simulink model "decimation"  (R2013b)
settings: Solver=ode45  StartTime=0.0  StopTime=10.0  RelTol=1e-3
undefined symbols (not defined in the file): xlfda_numerator
libraries: xbsIndex_r4 x1962, xps_library x2, casper_library_misc x1
(part 6 of 19)

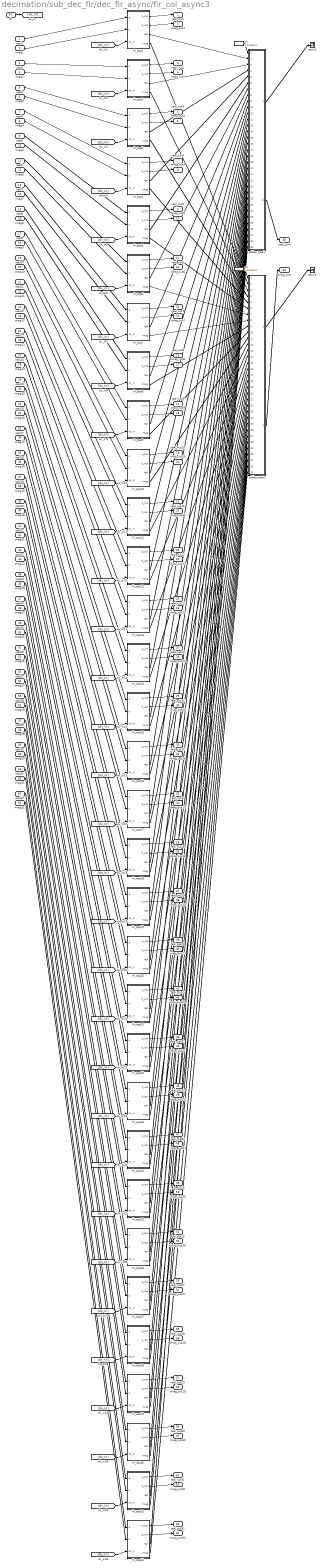
== system decimation/sub_dec_fir/dec_fir_async/fir_col_async3 ==
  real1 : Inport
  imag1 : Inport  Port=2
  real2 : Inport  Port=3
  imag2 : Inport  Port=4
  real3 : Inport  Port=5
  imag3 : Inport  Port=6
  real4 : Inport  Port=7
  imag4 : Inport  Port=8
  real5 : Inport  Port=9
  imag5 : Inport  Port=10
  real6 : Inport  Port=11
  imag6 : Inport  Port=12
  real7 : Inport  Port=13
  imag7 : Inport  Port=14
  real8 : Inport  Port=15
  imag8 : Inport  Port=16
  real9 : Inport  Port=17
  imag9 : Inport  Port=18
  real10 : Inport  Port=19
  imag10 : Inport  Port=20
  real11 : Inport  Port=21
  imag11 : Inport  Port=22
  real12 : Inport  Port=23
  imag12 : Inport  Port=24
  real13 : Inport  Port=25
  imag13 : Inport  Port=26
  real14 : Inport  Port=27
  imag14 : Inport  Port=28
  real15 : Inport  Port=29
  imag15 : Inport  Port=30
  real16 : Inport  Port=31
  imag16 : Inport  Port=32
  real17 : Inport  Port=33
  imag17 : Inport  Port=34
  real18 : Inport  Port=35
  imag18 : Inport  Port=36
  real19 : Inport  Port=37
  imag19 : Inport  Port=38
  real20 : Inport  Port=39
  imag20 : Inport  Port=40
  real21 : Inport  Port=41
  imag21 : Inport  Port=42
  real22 : Inport  Port=43
  imag22 : Inport  Port=44
  real23 : Inport  Port=45
  imag23 : Inport  Port=46
  real24 : Inport  Port=47
  imag24 : Inport  Port=48
  real25 : Inport  Port=49
  imag25 : Inport  Port=50
  real26 : Inport  Port=51
  imag26 : Inport  Port=52
  real27 : Inport  Port=53
  imag27 : Inport  Port=54
  real28 : Inport  Port=55
  imag28 : Inport  Port=56
  real29 : Inport  Port=57
  imag29 : Inport  Port=58
  real30 : Inport  Port=59
  imag30 : Inport  Port=60
  real31 : Inport  Port=61
  imag31 : Inport  Port=62
  real32 : Inport  Port=63
  imag32 : Inport  Port=64
  dv : Inport  Port=65
  adder_tree1 : Subsystem  AncestorBlock=casper_library_misc/adder_tree  mask(adder_tree){n_inputs=32, latency=1, adder_imp=DSP48, first_stage_hdl=on}
      mask prompts: n_inputs "Number of Inputs"; latency "Add Latency"; adder_imp "Adder implementation"; first_stage_hdl "Use behavioural HDL for first stage of adders"
      mask help:
      | Sums all inputs using a tree of adds and delays.
      |
      | Number of inputs: The number of inputs to the block to be summed
      | Add latency: The number of clock cycles to perform one addition (affects timing)..
      | Adder implementation: choice of fabric or DSP48E core, or behavioral HDL
      | Use behavioural HDL for first stage of adders: Causes the first stage of adders to be absorbed into DSP blocks if multipliers precede them (Virtex 5). Overrides Adder implementation
      mask init:
      | adder_tree_init(gcb, ...
      |     'n_inputs', n_inputs, ...
      |     'latency', latency, ...
      |     'adder_imp', adder_imp, ...
      |     'first_stage_hdl', first_stage_hdl);
      settings: AttributesFormatString=latency 5
      mask Help: eval('xlWeb(''http://casper.berkeley.edu/wiki/Adder_tree'')')
      mask TypeOptions adder_imp: Behavioral | Fabric | DSP48
  adder_tree2 : Subsystem  AncestorBlock=casper_library_misc/adder_tree  mask(adder_tree){n_inputs=32, latency=1, adder_imp=DSP48, first_stage_hdl=on}
      mask prompts: n_inputs "Number of Inputs"; latency "Add Latency"; adder_imp "Adder implementation"; first_stage_hdl "Use behavioural HDL for first stage of adders"
      mask help:
      | Sums all inputs using a tree of adds and delays.
      |
      | Number of inputs: The number of inputs to the block to be summed
      | Add latency: The number of clock cycles to perform one addition (affects timing)..
      | Adder implementation: choice of fabric or DSP48E core, or behavioral HDL
      | Use behavioural HDL for first stage of adders: Causes the first stage of adders to be absorbed into DSP blocks if multipliers precede them (Virtex 5). Overrides Adder implementation
      mask init:
      | adder_tree_init(gcb, ...
      |     'n_inputs', n_inputs, ...
      |     'latency', latency, ...
      |     'adder_imp', adder_imp, ...
      |     'first_stage_hdl', first_stage_hdl);
      settings: AttributesFormatString=latency 5
      mask Help: eval('xlWeb(''http://casper.berkeley.edu/wiki/Adder_tree'')')
      mask TypeOptions adder_imp: Behavioral | Fabric | DSP48
  c1 : xbsIndex_r4/Constant  const=1  gui_display_data_type=Fixed-point  arith_type=Signed (2's comp)  n_bits=16  bin_pt=14  preci_type=Single  exp_width=8  frac_width=24  explicit_period=on  period=1  equ=P=C  opselect=C  inp2=PCIN>>17  opr=+  inp1=P  carry=CIN  dbl_ovrd=off  block_type=constant
  c2 : xbsIndex_r4/Constant  const=1  gui_display_data_type=Fixed-point  arith_type=Signed (2's comp)  n_bits=16  bin_pt=14  preci_type=Single  exp_width=8  frac_width=24  explicit_period=on  period=1  equ=P=C  opselect=C  inp2=PCIN>>17  opr=+  inp1=P  carry=CIN  dbl_ovrd=off  block_type=constant
  fir_tap1 : Subsystem  AncestorBlock=casper_library_downconverter/fir_tap_async  mask(fir_tap_async){factor=-0.015819, add_latency=1, mult_latency=2, coeff_bit_width=25, coeff_bin_pt=24, async=on, dbl=off}
      mask prompts: add_latency "Add latency"; mult_latency "Mult latency"; coeff_bit_width "Coefficient bit width"; coeff_bin_pt "Coefficient binary point"; async "Asynchronous ops"; dbl "Double tap"
      mask help: Multiplies input data with factor specified.
      mask init:
      | fir_tap_async_init(gcb);
      mask Help: eval('xlWeb(''http://casper.berkeley.edu/wiki/Fir_tap'')')
  fir_tap10 : Subsystem  AncestorBlock=casper_library_downconverter/fir_tap_async  mask(fir_tap_async){factor=-0.0079781, add_latency=1, mult_latency=2, coeff_bit_width=25, coeff_bin_pt=24, async=on, dbl=off}
      mask prompts: add_latency "Add latency"; mult_latency "Mult latency"; coeff_bit_width "Coefficient bit width"; coeff_bin_pt "Coefficient binary point"; async "Asynchronous ops"; dbl "Double tap"
      mask help: Multiplies input data with factor specified.
      mask init:
      | fir_tap_async_init(gcb);
      mask Help: eval('xlWeb(''http://casper.berkeley.edu/wiki/Fir_tap'')')
  fir_tap11 : Subsystem  AncestorBlock=casper_library_downconverter/fir_tap_async  mask(fir_tap_async){factor=-0.0008307, add_latency=1, mult_latency=2, coeff_bit_width=25, coeff_bin_pt=24, async=on, dbl=off}
      mask prompts: add_latency "Add latency"; mult_latency "Mult latency"; coeff_bit_width "Coefficient bit width"; coeff_bin_pt "Coefficient binary point"; async "Asynchronous ops"; dbl "Double tap"
      mask help: Multiplies input data with factor specified.
      mask init:
      | fir_tap_async_init(gcb);
      mask Help: eval('xlWeb(''http://casper.berkeley.edu/wiki/Fir_tap'')')
  fir_tap12 : Subsystem  AncestorBlock=casper_library_downconverter/fir_tap_async  mask(fir_tap_async){factor=0.0066367, add_latency=1, mult_latency=2, coeff_bit_width=25, coeff_bin_pt=24, async=on, dbl=off}
      mask prompts: add_latency "Add latency"; mult_latency "Mult latency"; coeff_bit_width "Coefficient bit width"; coeff_bin_pt "Coefficient binary point"; async "Asynchronous ops"; dbl "Double tap"
      mask help: Multiplies input data with factor specified.
      mask init:
      | fir_tap_async_init(gcb);
      mask Help: eval('xlWeb(''http://casper.berkeley.edu/wiki/Fir_tap'')')
  fir_tap13 : Subsystem  AncestorBlock=casper_library_downconverter/fir_tap_async  mask(fir_tap_async){factor=0.0025836, add_latency=1, mult_latency=2, coeff_bit_width=25, coeff_bin_pt=24, async=on, dbl=off}
      mask prompts: add_latency "Add latency"; mult_latency "Mult latency"; coeff_bit_width "Coefficient bit width"; coeff_bin_pt "Coefficient binary point"; async "Asynchronous ops"; dbl "Double tap"
      mask help: Multiplies input data with factor specified.
      mask init:
      | fir_tap_async_init(gcb);
      mask Help: eval('xlWeb(''http://casper.berkeley.edu/wiki/Fir_tap'')')
  fir_tap14 : Subsystem  AncestorBlock=casper_library_downconverter/fir_tap_async  mask(fir_tap_async){factor=-0.0049848, add_latency=1, mult_latency=2, coeff_bit_width=25, coeff_bin_pt=24, async=on, dbl=off}
      mask prompts: add_latency "Add latency"; mult_latency "Mult latency"; coeff_bit_width "Coefficient bit width"; coeff_bin_pt "Coefficient binary point"; async "Asynchronous ops"; dbl "Double tap"
      mask help: Multiplies input data with factor specified.
      mask init:
      | fir_tap_async_init(gcb);
      mask Help: eval('xlWeb(''http://casper.berkeley.edu/wiki/Fir_tap'')')
  fir_tap15 : Subsystem  AncestorBlock=casper_library_downconverter/fir_tap_async  mask(fir_tap_async){factor=-0.0036243, add_latency=1, mult_latency=2, coeff_bit_width=25, coeff_bin_pt=24, async=on, dbl=off}
      mask prompts: add_latency "Add latency"; mult_latency "Mult latency"; coeff_bit_width "Coefficient bit width"; coeff_bin_pt "Coefficient binary point"; async "Asynchronous ops"; dbl "Double tap"
      mask help: Multiplies input data with factor specified.
      mask init:
      | fir_tap_async_init(gcb);
      mask Help: eval('xlWeb(''http://casper.berkeley.edu/wiki/Fir_tap'')')
  fir_tap16 : Subsystem  AncestorBlock=casper_library_downconverter/fir_tap_async  mask(fir_tap_async){factor=0.0032652, add_latency=1, mult_latency=2, coeff_bit_width=25, coeff_bin_pt=24, async=on, dbl=off}
      mask prompts: add_latency "Add latency"; mult_latency "Mult latency"; coeff_bit_width "Coefficient bit width"; coeff_bin_pt "Coefficient binary point"; async "Asynchronous ops"; dbl "Double tap"
      mask help: Multiplies input data with factor specified.
      mask init:
      | fir_tap_async_init(gcb);
      mask Help: eval('xlWeb(''http://casper.berkeley.edu/wiki/Fir_tap'')')
  fir_tap17 : Subsystem  AncestorBlock=casper_library_downconverter/fir_tap_async  mask(fir_tap_async){factor=0.0040292, add_latency=1, mult_latency=2, coeff_bit_width=25, coeff_bin_pt=24, async=on, dbl=off}
      mask prompts: add_latency "Add latency"; mult_latency "Mult latency"; coeff_bit_width "Coefficient bit width"; coeff_bin_pt "Coefficient binary point"; async "Asynchronous ops"; dbl "Double tap"
      mask help: Multiplies input data with factor specified.
      mask init:
      | fir_tap_async_init(gcb);
      mask Help: eval('xlWeb(''http://casper.berkeley.edu/wiki/Fir_tap'')')
  fir_tap18 : Subsystem  AncestorBlock=casper_library_downconverter/fir_tap_async  mask(fir_tap_async){factor=-0.0016691, add_latency=1, mult_latency=2, coeff_bit_width=25, coeff_bin_pt=24, async=on, dbl=off}
      mask prompts: add_latency "Add latency"; mult_latency "Mult latency"; coeff_bit_width "Coefficient bit width"; coeff_bin_pt "Coefficient binary point"; async "Asynchronous ops"; dbl "Double tap"
      mask help: Multiplies input data with factor specified.
      mask init:
      | fir_tap_async_init(gcb);
      mask Help: eval('xlWeb(''http://casper.berkeley.edu/wiki/Fir_tap'')')
  fir_tap19 : Subsystem  AncestorBlock=casper_library_downconverter/fir_tap_async  mask(fir_tap_async){factor=-0.0039196, add_latency=1, mult_latency=2, coeff_bit_width=25, coeff_bin_pt=24, async=on, dbl=off}
      mask prompts: add_latency "Add latency"; mult_latency "Mult latency"; coeff_bit_width "Coefficient bit width"; coeff_bin_pt "Coefficient binary point"; async "Asynchronous ops"; dbl "Double tap"
      mask help: Multiplies input data with factor specified.
      mask init:
      | fir_tap_async_init(gcb);
      mask Help: eval('xlWeb(''http://casper.berkeley.edu/wiki/Fir_tap'')')
  fir_tap2 : Subsystem  AncestorBlock=casper_library_downconverter/fir_tap_async  mask(fir_tap_async){factor=-0.0045283, add_latency=1, mult_latency=2, coeff_bit_width=25, coeff_bin_pt=24, async=on, dbl=off}
      mask prompts: add_latency "Add latency"; mult_latency "Mult latency"; coeff_bit_width "Coefficient bit width"; coeff_bin_pt "Coefficient binary point"; async "Asynchronous ops"; dbl "Double tap"
      mask help: Multiplies input data with factor specified.
      mask init:
      | fir_tap_async_init(gcb);
      mask Help: eval('xlWeb(''http://casper.berkeley.edu/wiki/Fir_tap'')')
  fir_tap20 : Subsystem  AncestorBlock=casper_library_downconverter/fir_tap_async  mask(fir_tap_async){factor=0.00032909, add_latency=1, mult_latency=2, coeff_bit_width=25, coeff_bin_pt=24, async=on, dbl=off}
      mask prompts: add_latency "Add latency"; mult_latency "Mult latency"; coeff_bit_width "Coefficient bit width"; coeff_bin_pt "Coefficient binary point"; async "Asynchronous ops"; dbl "Double tap"
      mask help: Multiplies input data with factor specified.
      mask init:
      | fir_tap_async_init(gcb);
      mask Help: eval('xlWeb(''http://casper.berkeley.edu/wiki/Fir_tap'')')
  fir_tap21 : Subsystem  AncestorBlock=casper_library_downconverter/fir_tap_async  mask(fir_tap_async){factor=0.0034399, add_latency=1, mult_latency=2, coeff_bit_width=25, coeff_bin_pt=24, async=on, dbl=off}
      mask prompts: add_latency "Add latency"; mult_latency "Mult latency"; coeff_bit_width "Coefficient bit width"; coeff_bin_pt "Coefficient binary point"; async "Asynchronous ops"; dbl "Double tap"
      mask help: Multiplies input data with factor specified.
      mask init:
      | fir_tap_async_init(gcb);
      mask Help: eval('xlWeb(''http://casper.berkeley.edu/wiki/Fir_tap'')')
  fir_tap22 : Subsystem  AncestorBlock=casper_library_downconverter/fir_tap_async  mask(fir_tap_async){factor=0.00068177, add_latency=1, mult_latency=2, coeff_bit_width=25, coeff_bin_pt=24, async=on, dbl=off}
      mask prompts: add_latency "Add latency"; mult_latency "Mult latency"; coeff_bit_width "Coefficient bit width"; coeff_bin_pt "Coefficient binary point"; async "Asynchronous ops"; dbl "Double tap"
      mask help: Multiplies input data with factor specified.
      mask init:
      | fir_tap_async_init(gcb);
      mask Help: eval('xlWeb(''http://casper.berkeley.edu/wiki/Fir_tap'')')
  fir_tap23 : Subsystem  AncestorBlock=casper_library_downconverter/fir_tap_async  mask(fir_tap_async){factor=-0.0027376, add_latency=1, mult_latency=2, coeff_bit_width=25, coeff_bin_pt=24, async=on, dbl=off}
      mask prompts: add_latency "Add latency"; mult_latency "Mult latency"; coeff_bit_width "Coefficient bit width"; coeff_bin_pt "Coefficient binary point"; async "Asynchronous ops"; dbl "Double tap"
      mask help: Multiplies input data with factor specified.
      mask init:
      | fir_tap_async_init(gcb);
      mask Help: eval('xlWeb(''http://casper.berkeley.edu/wiki/Fir_tap'')')
  fir_tap24 : Subsystem  AncestorBlock=casper_library_downconverter/fir_tap_async  mask(fir_tap_async){factor=-0.0013435, add_latency=1, mult_latency=2, coeff_bit_width=25, coeff_bin_pt=24, async=on, dbl=off}
      mask prompts: add_latency "Add latency"; mult_latency "Mult latency"; coeff_bit_width "Coefficient bit width"; coeff_bin_pt "Coefficient binary point"; async "Asynchronous ops"; dbl "Double tap"
      mask help: Multiplies input data with factor specified.
      mask init:
      | fir_tap_async_init(gcb);
      mask Help: eval('xlWeb(''http://casper.berkeley.edu/wiki/Fir_tap'')')
  fir_tap25 : Subsystem  AncestorBlock=casper_library_downconverter/fir_tap_async  mask(fir_tap_async){factor=0.0019468, add_latency=1, mult_latency=2, coeff_bit_width=25, coeff_bin_pt=24, async=on, dbl=off}
      mask prompts: add_latency "Add latency"; mult_latency "Mult latency"; coeff_bit_width "Coefficient bit width"; coeff_bin_pt "Coefficient binary point"; async "Asynchronous ops"; dbl "Double tap"
      mask help: Multiplies input data with factor specified.
      mask init:
      | fir_tap_async_init(gcb);
      mask Help: eval('xlWeb(''http://casper.berkeley.edu/wiki/Fir_tap'')')
  fir_tap26 : Subsystem  AncestorBlock=casper_library_downconverter/fir_tap_async  mask(fir_tap_async){factor=0.0016792, add_latency=1, mult_latency=2, coeff_bit_width=25, coeff_bin_pt=24, async=on, dbl=off}
      mask prompts: add_latency "Add latency"; mult_latency "Mult latency"; coeff_bit_width "Coefficient bit width"; coeff_bin_pt "Coefficient binary point"; async "Asynchronous ops"; dbl "Double tap"
      mask help: Multiplies input data with factor specified.
      mask init:
      | fir_tap_async_init(gcb);
      mask Help: eval('xlWeb(''http://casper.berkeley.edu/wiki/Fir_tap'')')
  fir_tap27 : Subsystem  AncestorBlock=casper_library_downconverter/fir_tap_async  mask(fir_tap_async){factor=-0.0011769, add_latency=1, mult_latency=2, coeff_bit_width=25, coeff_bin_pt=24, async=on, dbl=off}
      mask prompts: add_latency "Add latency"; mult_latency "Mult latency"; coeff_bit_width "Coefficient bit width"; coeff_bin_pt "Coefficient binary point"; async "Asynchronous ops"; dbl "Double tap"
      mask help: Multiplies input data with factor specified.
      mask init:
      | fir_tap_async_init(gcb);
      mask Help: eval('xlWeb(''http://casper.berkeley.edu/wiki/Fir_tap'')')
  fir_tap28 : Subsystem  AncestorBlock=casper_library_downconverter/fir_tap_async  mask(fir_tap_async){factor=-0.0017418, add_latency=1, mult_latency=2, coeff_bit_width=25, coeff_bin_pt=24, async=on, dbl=off}
      mask prompts: add_latency "Add latency"; mult_latency "Mult latency"; coeff_bit_width "Coefficient bit width"; coeff_bin_pt "Coefficient binary point"; async "Asynchronous ops"; dbl "Double tap"
      mask help: Multiplies input data with factor specified.
      mask init:
      | fir_tap_async_init(gcb);
      mask Help: eval('xlWeb(''http://casper.berkeley.edu/wiki/Fir_tap'')')
  fir_tap29 : Subsystem  AncestorBlock=casper_library_downconverter/fir_tap_async  mask(fir_tap_async){factor=0.00050609, add_latency=1, mult_latency=2, coeff_bit_width=25, coeff_bin_pt=24, async=on, dbl=off}
      mask prompts: add_latency "Add latency"; mult_latency "Mult latency"; coeff_bit_width "Coefficient bit width"; coeff_bin_pt "Coefficient binary point"; async "Asynchronous ops"; dbl "Double tap"
      mask help: Multiplies input data with factor specified.
      mask init:
      | fir_tap_async_init(gcb);
      mask Help: eval('xlWeb(''http://casper.berkeley.edu/wiki/Fir_tap'')')
  fir_tap3 : Subsystem  AncestorBlock=casper_library_downconverter/fir_tap_async  mask(fir_tap_async){factor=0.012178, add_latency=1, mult_latency=2, coeff_bit_width=25, coeff_bin_pt=24, async=on, dbl=off}
      mask prompts: add_latency "Add latency"; mult_latency "Mult latency"; coeff_bit_width "Coefficient bit width"; coeff_bin_pt "Coefficient binary point"; async "Asynchronous ops"; dbl "Double tap"
      mask help: Multiplies input data with factor specified.
      mask init:
      | fir_tap_async_init(gcb);
      mask Help: eval('xlWeb(''http://casper.berkeley.edu/wiki/Fir_tap'')')
  fir_tap30 : Subsystem  AncestorBlock=casper_library_downconverter/fir_tap_async  mask(fir_tap_async){factor=0.0016008, add_latency=1, mult_latency=2, coeff_bit_width=25, coeff_bin_pt=24, async=on, dbl=off}
      mask prompts: add_latency "Add latency"; mult_latency "Mult latency"; coeff_bit_width "Coefficient bit width"; coeff_bin_pt "Coefficient binary point"; async "Asynchronous ops"; dbl "Double tap"
      mask help: Multiplies input data with factor specified.
      mask init:
      | fir_tap_async_init(gcb);
      mask Help: eval('xlWeb(''http://casper.berkeley.edu/wiki/Fir_tap'')')
  fir_tap31 : Subsystem  AncestorBlock=casper_library_downconverter/fir_tap_async  mask(fir_tap_async){factor=1.9493e-05, add_latency=1, mult_latency=2, coeff_bit_width=25, coeff_bin_pt=24, async=on, dbl=off}
      mask prompts: add_latency "Add latency"; mult_latency "Mult latency"; coeff_bit_width "Coefficient bit width"; coeff_bin_pt "Coefficient binary point"; async "Asynchronous ops"; dbl "Double tap"
      mask help: Multiplies input data with factor specified.
      mask init:
      | fir_tap_async_init(gcb);
      mask Help: eval('xlWeb(''http://casper.berkeley.edu/wiki/Fir_tap'')')
  fir_tap32 : Subsystem  AncestorBlock=casper_library_downconverter/fir_tap_async  mask(fir_tap_async){factor=-0.0013302, add_latency=1, mult_latency=2, coeff_bit_width=25, coeff_bin_pt=24, async=on, dbl=off}
      mask prompts: add_latency "Add latency"; mult_latency "Mult latency"; coeff_bit_width "Coefficient bit width"; coeff_bin_pt "Coefficient binary point"; async "Asynchronous ops"; dbl "Double tap"
      mask help: Multiplies input data with factor specified.
      mask init:
      | fir_tap_async_init(gcb);
      mask Help: eval('xlWeb(''http://casper.berkeley.edu/wiki/Fir_tap'')')
  fir_tap4 : Subsystem  AncestorBlock=casper_library_downconverter/fir_tap_async  mask(fir_tap_async){factor=0.0072795, add_latency=1, mult_latency=2, coeff_bit_width=25, coeff_bin_pt=24, async=on, dbl=off}
      mask prompts: add_latency "Add latency"; mult_latency "Mult latency"; coeff_bit_width "Coefficient bit width"; coeff_bin_pt "Coefficient binary point"; async "Asynchronous ops"; dbl "Double tap"
      mask help: Multiplies input data with factor specified.
      mask init:
      | fir_tap_async_init(gcb);
      mask Help: eval('xlWeb(''http://casper.berkeley.edu/wiki/Fir_tap'')')
  fir_tap5 : Subsystem  AncestorBlock=casper_library_downconverter/fir_tap_async  mask(fir_tap_async){factor=-0.0083697, add_latency=1, mult_latency=2, coeff_bit_width=25, coeff_bin_pt=24, async=on, dbl=off}
      mask prompts: add_latency "Add latency"; mult_latency "Mult latency"; coeff_bit_width "Coefficient bit width"; coeff_bin_pt "Coefficient binary point"; async "Asynchronous ops"; dbl "Double tap"
      mask help: Multiplies input data with factor specified.
      mask init:
      | fir_tap_async_init(gcb);
      mask Help: eval('xlWeb(''http://casper.berkeley.edu/wiki/Fir_tap'')')
  fir_tap6 : Subsystem  AncestorBlock=casper_library_downconverter/fir_tap_async  mask(fir_tap_async){factor=-0.0085928, add_latency=1, mult_latency=2, coeff_bit_width=25, coeff_bin_pt=24, async=on, dbl=off}
      mask prompts: add_latency "Add latency"; mult_latency "Mult latency"; coeff_bit_width "Coefficient bit width"; coeff_bin_pt "Coefficient binary point"; async "Asynchronous ops"; dbl "Double tap"
      mask help: Multiplies input data with factor specified.
      mask init:
      | fir_tap_async_init(gcb);
      mask Help: eval('xlWeb(''http://casper.berkeley.edu/wiki/Fir_tap'')')
  fir_tap7 : Subsystem  AncestorBlock=casper_library_downconverter/fir_tap_async  mask(fir_tap_async){factor=0.004768, add_latency=1, mult_latency=2, coeff_bit_width=25, coeff_bin_pt=24, async=on, dbl=off}
      mask prompts: add_latency "Add latency"; mult_latency "Mult latency"; coeff_bit_width "Coefficient bit width"; coeff_bin_pt "Coefficient binary point"; async "Asynchronous ops"; dbl "Double tap"
      mask help: Multiplies input data with factor specified.
      mask init:
      | fir_tap_async_init(gcb);
      mask Help: eval('xlWeb(''http://casper.berkeley.edu/wiki/Fir_tap'')')
  fir_tap8 : Subsystem  AncestorBlock=casper_library_downconverter/fir_tap_async  mask(fir_tap_async){factor=0.008729, add_latency=1, mult_latency=2, coeff_bit_width=25, coeff_bin_pt=24, async=on, dbl=off}
      mask prompts: add_latency "Add latency"; mult_latency "Mult latency"; coeff_bit_width "Coefficient bit width"; coeff_bin_pt "Coefficient binary point"; async "Asynchronous ops"; dbl "Double tap"
      mask help: Multiplies input data with factor specified.
      mask init:
      | fir_tap_async_init(gcb);
      mask Help: eval('xlWeb(''http://casper.berkeley.edu/wiki/Fir_tap'')')
  fir_tap9 : Subsystem  AncestorBlock=casper_library_downconverter/fir_tap_async  mask(fir_tap_async){factor=-0.0016445, add_latency=1, mult_latency=2, coeff_bit_width=25, coeff_bin_pt=24, async=on, dbl=off}
      mask prompts: add_latency "Add latency"; mult_latency "Mult latency"; coeff_bit_width "Coefficient bit width"; coeff_bin_pt "Coefficient binary point"; async "Asynchronous ops"; dbl "Double tap"
      mask help: Multiplies input data with factor specified.
      mask init:
      | fir_tap_async_init(gcb);
      mask Help: eval('xlWeb(''http://casper.berkeley.edu/wiki/Fir_tap'')')
  term1 : Terminator
  term2 : Terminator
  real_out1 : Outport
  imag_out1 : Outport  Port=2
  real_out2 : Outport  Port=3
  imag_out2 : Outport  Port=4
  real_out3 : Outport  Port=5
  imag_out3 : Outport  Port=6
  real_out4 : Outport  Port=7
  imag_out4 : Outport  Port=8
  real_out5 : Outport  Port=9
  imag_out5 : Outport  Port=10
  real_out6 : Outport  Port=11
  imag_out6 : Outport  Port=12
  real_out7 : Outport  Port=13
  imag_out7 : Outport  Port=14
  real_out8 : Outport  Port=15
  imag_out8 : Outport  Port=16
  real_out9 : Outport  Port=17
  imag_out9 : Outport  Port=18
  real_out10 : Outport  Port=19
  imag_out10 : Outport  Port=20
  real_out11 : Outport  Port=21
  imag_out11 : Outport  Port=22
  real_out12 : Outport  Port=23
  imag_out12 : Outport  Port=24
  real_out13 : Outport  Port=25
  imag_out13 : Outport  Port=26
  real_out14 : Outport  Port=27
  imag_out14 : Outport  Port=28
  real_out15 : Outport  Port=29
  imag_out15 : Outport  Port=30
  real_out16 : Outport  Port=31
  imag_out16 : Outport  Port=32
  real_out17 : Outport  Port=33
  imag_out17 : Outport  Port=34
  real_out18 : Outport  Port=35
  imag_out18 : Outport  Port=36
  real_out19 : Outport  Port=37
  imag_out19 : Outport  Port=38
  real_out20 : Outport  Port=39
  imag_out20 : Outport  Port=40
  real_out21 : Outport  Port=41
  imag_out21 : Outport  Port=42
  real_out22 : Outport  Port=43
  imag_out22 : Outport  Port=44
  real_out23 : Outport  Port=45
  imag_out23 : Outport  Port=46
  real_out24 : Outport  Port=47
  imag_out24 : Outport  Port=48
  real_out25 : Outport  Port=49
  imag_out25 : Outport  Port=50
  real_out26 : Outport  Port=51
  imag_out26 : Outport  Port=52
  real_out27 : Outport  Port=53
  imag_out27 : Outport  Port=54
  real_out28 : Outport  Port=55
  imag_out28 : Outport  Port=56
  real_out29 : Outport  Port=57
  imag_out29 : Outport  Port=58
  real_out30 : Outport  Port=59
  imag_out30 : Outport  Port=60
  real_out31 : Outport  Port=61
  imag_out31 : Outport  Port=62
  real_out32 : Outport  Port=63
  imag_out32 : Outport  Port=64
  real_sum : Outport  Port=65
  imag_sum : Outport  Port=66
  wires:
  dv/1 -> [dv_in]
  [dv_in] -> fir_tap1/3(dv_in)
  real1/1 -> fir_tap1/1(a)
  imag1/1 -> fir_tap1/2(b)
  [dv_in] -> fir_tap2/3(dv_in)
  real2/1 -> fir_tap2/1(a)
  imag2/1 -> fir_tap2/2(b)
  [dv_in] -> fir_tap3/3(dv_in)
  real3/1 -> fir_tap3/1(a)
  imag3/1 -> fir_tap3/2(b)
  [dv_in] -> fir_tap4/3(dv_in)
  real4/1 -> fir_tap4/1(a)
  imag4/1 -> fir_tap4/2(b)
  [dv_in] -> fir_tap5/3(dv_in)
  real5/1 -> fir_tap5/1(a)
  imag5/1 -> fir_tap5/2(b)
  [dv_in] -> fir_tap6/3(dv_in)
  real6/1 -> fir_tap6/1(a)
  imag6/1 -> fir_tap6/2(b)
  [dv_in] -> fir_tap7/3(dv_in)
  real7/1 -> fir_tap7/1(a)
  imag7/1 -> fir_tap7/2(b)
  [dv_in] -> fir_tap8/3(dv_in)
  real8/1 -> fir_tap8/1(a)
  imag8/1 -> fir_tap8/2(b)
  [dv_in] -> fir_tap9/3(dv_in)
  real9/1 -> fir_tap9/1(a)
  imag9/1 -> fir_tap9/2(b)
  [dv_in] -> fir_tap10/3(dv_in)
  real10/1 -> fir_tap10/1(a)
  imag10/1 -> fir_tap10/2(b)
  [dv_in] -> fir_tap11/3(dv_in)
  real11/1 -> fir_tap11/1(a)
  imag11/1 -> fir_tap11/2(b)
  [dv_in] -> fir_tap12/3(dv_in)
  real12/1 -> fir_tap12/1(a)
  imag12/1 -> fir_tap12/2(b)
  [dv_in] -> fir_tap13/3(dv_in)
  real13/1 -> fir_tap13/1(a)
  imag13/1 -> fir_tap13/2(b)
  [dv_in] -> fir_tap14/3(dv_in)
  real14/1 -> fir_tap14/1(a)
  imag14/1 -> fir_tap14/2(b)
  [dv_in] -> fir_tap15/3(dv_in)
  real15/1 -> fir_tap15/1(a)
  imag15/1 -> fir_tap15/2(b)
  [dv_in] -> fir_tap16/3(dv_in)
  real16/1 -> fir_tap16/1(a)
  imag16/1 -> fir_tap16/2(b)
  [dv_in] -> fir_tap17/3(dv_in)
  real17/1 -> fir_tap17/1(a)
  imag17/1 -> fir_tap17/2(b)
  [dv_in] -> fir_tap18/3(dv_in)
  real18/1 -> fir_tap18/1(a)
  imag18/1 -> fir_tap18/2(b)
  [dv_in] -> fir_tap19/3(dv_in)
  real19/1 -> fir_tap19/1(a)
  imag19/1 -> fir_tap19/2(b)
  [dv_in] -> fir_tap20/3(dv_in)
  real20/1 -> fir_tap20/1(a)
  imag20/1 -> fir_tap20/2(b)
  [dv_in] -> fir_tap21/3(dv_in)
  real21/1 -> fir_tap21/1(a)
  imag21/1 -> fir_tap21/2(b)
  [dv_in] -> fir_tap22/3(dv_in)
  real22/1 -> fir_tap22/1(a)
  imag22/1 -> fir_tap22/2(b)
  [dv_in] -> fir_tap23/3(dv_in)
  real23/1 -> fir_tap23/1(a)
  imag23/1 -> fir_tap23/2(b)
  [dv_in] -> fir_tap24/3(dv_in)
  real24/1 -> fir_tap24/1(a)
  imag24/1 -> fir_tap24/2(b)
  [dv_in] -> fir_tap25/3(dv_in)
  real25/1 -> fir_tap25/1(a)
  imag25/1 -> fir_tap25/2(b)
  [dv_in] -> fir_tap26/3(dv_in)
  real26/1 -> fir_tap26/1(a)
  imag26/1 -> fir_tap26/2(b)
  [dv_in] -> fir_tap27/3(dv_in)
  real27/1 -> fir_tap27/1(a)
  imag27/1 -> fir_tap27/2(b)
  [dv_in] -> fir_tap28/3(dv_in)
  real28/1 -> fir_tap28/1(a)
  imag28/1 -> fir_tap28/2(b)
  [dv_in] -> fir_tap29/3(dv_in)
  real29/1 -> fir_tap29/1(a)
  imag29/1 -> fir_tap29/2(b)
  [dv_in] -> fir_tap30/3(dv_in)
  real30/1 -> fir_tap30/1(a)
  imag30/1 -> fir_tap30/2(b)
  [dv_in] -> fir_tap31/3(dv_in)
  real31/1 -> fir_tap31/1(a)
  imag31/1 -> fir_tap31/2(b)
  [dv_in] -> fir_tap32/3(dv_in)
  real32/1 -> fir_tap32/1(a)
  imag32/1 -> fir_tap32/2(b)
  fir_tap1/1(a_out) -> real_out1/1
  fir_tap1/2(b_out) -> imag_out1/1
  fir_tap2/1(a_out) -> real_out2/1
  fir_tap2/2(b_out) -> imag_out2/1
  fir_tap3/1(a_out) -> real_out3/1
  fir_tap3/2(b_out) -> imag_out3/1
  fir_tap4/1(a_out) -> real_out4/1
  fir_tap4/2(b_out) -> imag_out4/1
  fir_tap5/1(a_out) -> real_out5/1
  fir_tap5/2(b_out) -> imag_out5/1
  fir_tap6/1(a_out) -> real_out6/1
  fir_tap6/2(b_out) -> imag_out6/1
  fir_tap7/1(a_out) -> real_out7/1
  fir_tap7/2(b_out) -> imag_out7/1
  fir_tap8/1(a_out) -> real_out8/1
  fir_tap8/2(b_out) -> imag_out8/1
  fir_tap9/1(a_out) -> real_out9/1
  fir_tap9/2(b_out) -> imag_out9/1
  fir_tap10/1(a_out) -> real_out10/1
  fir_tap10/2(b_out) -> imag_out10/1
  fir_tap11/1(a_out) -> real_out11/1
  fir_tap11/2(b_out) -> imag_out11/1
  fir_tap12/1(a_out) -> real_out12/1
  fir_tap12/2(b_out) -> imag_out12/1
  fir_tap13/1(a_out) -> real_out13/1
  fir_tap13/2(b_out) -> imag_out13/1
  fir_tap14/1(a_out) -> real_out14/1
  fir_tap14/2(b_out) -> imag_out14/1
  fir_tap15/1(a_out) -> real_out15/1
  fir_tap15/2(b_out) -> imag_out15/1
  fir_tap16/1(a_out) -> real_out16/1
  fir_tap16/2(b_out) -> imag_out16/1
  fir_tap17/1(a_out) -> real_out17/1
  fir_tap17/2(b_out) -> imag_out17/1
  fir_tap18/1(a_out) -> real_out18/1
  fir_tap18/2(b_out) -> imag_out18/1
  fir_tap19/1(a_out) -> real_out19/1
  fir_tap19/2(b_out) -> imag_out19/1
  fir_tap20/1(a_out) -> real_out20/1
  fir_tap20/2(b_out) -> imag_out20/1
  fir_tap21/1(a_out) -> real_out21/1
  fir_tap21/2(b_out) -> imag_out21/1
  fir_tap22/1(a_out) -> real_out22/1
  fir_tap22/2(b_out) -> imag_out22/1
  fir_tap23/1(a_out) -> real_out23/1
  fir_tap23/2(b_out) -> imag_out23/1
  fir_tap24/1(a_out) -> real_out24/1
  fir_tap24/2(b_out) -> imag_out24/1
  fir_tap25/1(a_out) -> real_out25/1
  fir_tap25/2(b_out) -> imag_out25/1
  fir_tap26/1(a_out) -> real_out26/1
  fir_tap26/2(b_out) -> imag_out26/1
  fir_tap27/1(a_out) -> real_out27/1
  fir_tap27/2(b_out) -> imag_out27/1
  fir_tap28/1(a_out) -> real_out28/1
  fir_tap28/2(b_out) -> imag_out28/1
  fir_tap29/1(a_out) -> real_out29/1
  fir_tap29/2(b_out) -> imag_out29/1
  fir_tap30/1(a_out) -> real_out30/1
  fir_tap30/2(b_out) -> imag_out30/1
  fir_tap31/1(a_out) -> real_out31/1
  fir_tap31/2(b_out) -> imag_out31/1
  fir_tap32/1(a_out) -> real_out32/1
  fir_tap32/2(b_out) -> imag_out32/1
  adder_tree1/1(sync_out) -> term1/1
  adder_tree2/1(sync_out) -> term2/1
  c1/1 -> adder_tree1/1(sync)
  c2/1 -> adder_tree2/1(sync)
  adder_tree1/2(dout) -> real_sum/1
  adder_tree2/2(dout) -> imag_sum/1
  fir_tap1/3(real) -> adder_tree1/2(din1)
  fir_tap1/4(imag) -> adder_tree2/2(din1)
  fir_tap2/3(real) -> adder_tree1/3(din2)
  fir_tap2/4(imag) -> adder_tree2/3(din2)
  fir_tap3/3(real) -> adder_tree1/4(din3)
  fir_tap3/4(imag) -> adder_tree2/4(din3)
  fir_tap4/3(real) -> adder_tree1/5(din4)
  fir_tap4/4(imag) -> adder_tree2/5(din4)
  fir_tap5/3(real) -> adder_tree1/6(din5)
  fir_tap5/4(imag) -> adder_tree2/6(din5)
  fir_tap6/3(real) -> adder_tree1/7(din6)
  fir_tap6/4(imag) -> adder_tree2/7(din6)
  fir_tap7/3(real) -> adder_tree1/8(din7)
  fir_tap7/4(imag) -> adder_tree2/8(din7)
  fir_tap8/3(real) -> adder_tree1/9(din8)
  fir_tap8/4(imag) -> adder_tree2/9(din8)
  fir_tap9/3(real) -> adder_tree1/10(din9)
  fir_tap9/4(imag) -> adder_tree2/10(din9)
  fir_tap10/3(real) -> adder_tree1/11(din10)
  fir_tap10/4(imag) -> adder_tree2/11(din10)
  fir_tap11/3(real) -> adder_tree1/12(din11)
  fir_tap11/4(imag) -> adder_tree2/12(din11)
  fir_tap12/3(real) -> adder_tree1/13(din12)
  fir_tap12/4(imag) -> adder_tree2/13(din12)
  fir_tap13/3(real) -> adder_tree1/14(din13)
  fir_tap13/4(imag) -> adder_tree2/14(din13)
  fir_tap14/3(real) -> adder_tree1/15(din14)
  fir_tap14/4(imag) -> adder_tree2/15(din14)
  fir_tap15/3(real) -> adder_tree1/16(din15)
  fir_tap15/4(imag) -> adder_tree2/16(din15)
  fir_tap16/3(real) -> adder_tree1/17(din16)
  fir_tap16/4(imag) -> adder_tree2/17(din16)
  fir_tap17/3(real) -> adder_tree1/18(din17)
  fir_tap17/4(imag) -> adder_tree2/18(din17)
  fir_tap18/3(real) -> adder_tree1/19(din18)
  fir_tap18/4(imag) -> adder_tree2/19(din18)
  fir_tap19/3(real) -> adder_tree1/20(din19)
  fir_tap19/4(imag) -> adder_tree2/20(din19)
  fir_tap20/3(real) -> adder_tree1/21(din20)
  fir_tap20/4(imag) -> adder_tree2/21(din20)
  fir_tap21/3(real) -> adder_tree1/22(din21)
  fir_tap21/4(imag) -> adder_tree2/22(din21)
  fir_tap22/3(real) -> adder_tree1/23(din22)
  fir_tap22/4(imag) -> adder_tree2/23(din22)
  fir_tap23/3(real) -> adder_tree1/24(din23)
  fir_tap23/4(imag) -> adder_tree2/24(din23)
  fir_tap24/3(real) -> adder_tree1/25(din24)
  fir_tap24/4(imag) -> adder_tree2/25(din24)
  fir_tap25/3(real) -> adder_tree1/26(din25)
  fir_tap25/4(imag) -> adder_tree2/26(din25)
  fir_tap26/3(real) -> adder_tree1/27(din26)
  fir_tap26/4(imag) -> adder_tree2/27(din26)
  fir_tap27/3(real) -> adder_tree1/28(din27)
  fir_tap27/4(imag) -> adder_tree2/28(din27)
  fir_tap28/3(real) -> adder_tree1/29(din28)
  fir_tap28/4(imag) -> adder_tree2/29(din28)
  fir_tap29/3(real) -> adder_tree1/30(din29)
  fir_tap29/4(imag) -> adder_tree2/30(din29)
  fir_tap30/3(real) -> adder_tree1/31(din30)
  fir_tap30/4(imag) -> adder_tree2/31(din30)
  fir_tap31/3(real) -> adder_tree1/32(din31)
  fir_tap31/4(imag) -> adder_tree2/32(din31)
  fir_tap32/3(real) -> adder_tree1/33(din32)
  fir_tap32/4(imag) -> adder_tree2/33(din32)
